simulink model "CACC_system_struct"  (Simulink 8.2)
settings: Solver=ode1  SolverMode=SingleTasking  StartTime=0.0  StopTime=inf  FixedStep=0.01  RelTol=1e-3
PreLoadFcn:
  | numd_dvsp = [0.3579 0 -0.3579];
  | dend_dvsp = [1 -1.846 0.8535];
  | simpleacc_param
PostLoadFcn:
  | , if any(exist('dsrtsu_mdlpostloadfcn', 'file') == [2, 3, 6]), try dsrtsu_mdlpostloadfcn('Execute', bdroot); catch fprintf('Error in PostLoadFcn (dsrtsu_mdlpostloadfcn) for model "%s":\n %s\n', bdroot, lasterr); end, end,
undefined symbols (not defined in the file): command_mode, max_accel_m_s2, override_enabled, speed_command_m_s, wrench_effort_command
libraries: carma_platform x3, dsrc_transmitter x2, rtitttasklib x2, lightbar x2, srx_platform x1
(part 3 of 4)

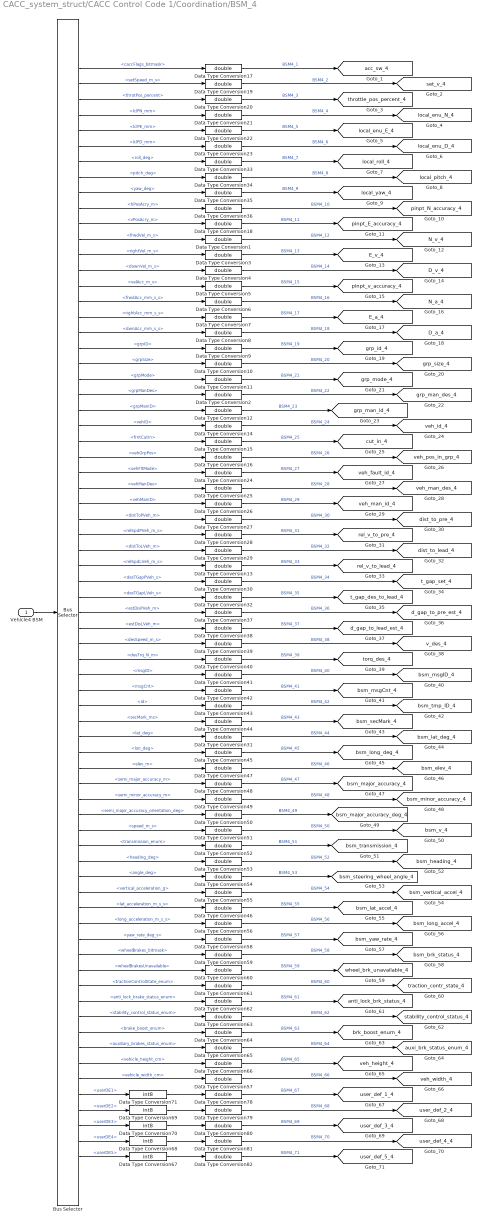
== system CACC_system_struct/CACC Control Code 1/Coordination/BSM_4 ==
  Vehicle4 BSM : Inport
  Bus Selector : BusSelector  OutputSignals=caccFlags_bitmask,setSpeed_m_s,throtPos_percent,lclPN_mm,lclPE_mm,lclPD_mm,roll_deg,pitch_deg,yaw_deg,hPosAcry_m,vPosAcry_m,frwdVel_m_s,rightVel_m_s,downVel_m_s,velAcc_m_s,frwdAcc_mm_s_s,rightAcc_mm_s_s,dwnAcc_mm_s_s,grpID,grpSize,grpMode,grpManDes,grpManID,vehID,frntCutIn,vehGrpPos,vehFltMode,vehManDes,vehManID,distToPVeh_m,relSpdPVeh_m_s,distToLVeh_m,relSpdLVeh_m_s,desTGapPVeh_s,desTGapLVeh_s,estDisPVeh_m,estDisLVeh_m,desSpeed_m_s,desTrq_N_m,msgID,msgCnt,id,secMark_ms,lat_deg,lon_deg,elev_m,semi_major_accuracy_m,semi_minor_accuracy_m,semi_major_accuracy_orientation_deg,speed_m_s,transmission_enum,heading_deg,angle_deg,vertical_acceleration_g,lat_acceleration_m_s_s,long_acceleration_m_s_s,yaw_rate_deg_s,wheelBrakes_bitmask,wheelBrakesUnavailable,tractionControlState_enum,anti_lock_brake_status_enum,stability_control_status_enum,brake_boost_enum,auxiliary_brakes_status_enum,vehicle_height_cm,vehicle_width_cm,userDE1,userDE2,userDE3,userDE4,userDE5
  Data Type Conversion{1..66,78..82} (71 alike) : DataTypeConversion  OutMin=[0]  OutMax=[5]  OutDataTypeStr=double
  Data Type Conversion{67..71} (5 alike) : DataTypeConversion  OutMin=[-128]  OutMax=[127]  OutDataTypeStr=int8  ConvertRealWorld=Stored Integer (SI)
  tag scope: D_a_4=global, D_v_4=global, E_a_4=global, E_v_4=global, N_a_4=global, N_v_4=global, acc_sw_4=global, anti_lock_brk_status_4=global, auxi_brk_status_enum_4=global, brk_boost_enum_4=global, bsm_brk_status_4=global, bsm_elev_4=global, bsm_heading_4=global, bsm_lat_accel_4=global, bsm_lat_deg_4=global, bsm_long_accel_4=global, bsm_long_deg_4=global, bsm_major_accuracy_4=global, bsm_major_accuracy_deg_4=global, bsm_minor_accuracy_4=global, bsm_msgCnt_4=global, bsm_msgID_4=global, bsm_secMark_4=global, bsm_steering_wheel_angle_4=global, bsm_tmp_ID_4=global, bsm_transmission_4=global, bsm_v_4=global, bsm_vertical_accel_4=global, bsm_yaw_rate_4=global, cut_in_4=global, d_gap_to_lead_est_4=global, d_gap_to_pre_est_4=global, dist_to_lead_4=global, dist_to_pre_4=global, grp_id_4=global, grp_man_des_4=global, grp_man_id_4=global, grp_mode_4=global, grp_size_4=global, local_enu_D_4=global, local_enu_E_4=global, local_enu_N_4=global, local_pitch_4=global, local_roll_4=global, local_yaw_4=global, pinpt_E_accuracy_4=global, pinpt_N_accuracy_4=global, pinpt_v_accuracy_4=global, rel_v_to_lead_4=global, rel_v_to_pre_4=global, set_v_4=global, stability_control_status_4=global, t_gap_des_to_lead_4=global, t_gap_set_4=global, throttle_pos_percent_4=global, torq_des_4=global, traction_contr_state_4=global, user_def_1_4=global, user_def_2_4=global, user_def_3_4=global, user_def_4_4=global, user_def_5_4=global, v_des_4=global, veh_fault_id_4=global, veh_height_4=global, veh_id_4=global, veh_man_des_4=global, veh_man_id_4=global, veh_pos_in_grp_4=global, veh_width_4=global, wheel_brk_unavailable_4=global
  wires:
  Vehicle4 BSM/1 -> Bus Selector/1
  Bus Selector/34 -> Data Type Conversion30/1  "<desTGapPVeh_s>"
  Bus Selector/33 -> Data Type Conversion13/1  "<relSpdLVeh_m_s>"
  Bus Selector/2 -> Data Type Conversion19/1  "<setSpeed_m_s>"
  Bus Selector/1 -> Data Type Conversion17/1  "<caccFlags_bitmask>"
  Bus Selector/7 -> Data Type Conversion33/1  "<roll_deg>"
  Bus Selector/3 -> Data Type Conversion20/1  "<throtPos_percent>"
  Bus Selector/9 -> Data Type Conversion35/1  "<yaw_deg>"
  Bus Selector/8 -> Data Type Conversion34/1  "<pitch_deg>"
  Bus Selector/11 -> Data Type Conversion18/1  "<vPosAcry_m>"
  Bus Selector/10 -> Data Type Conversion36/1  "<hPosAcry_m>"
  Bus Selector/13 -> Data Type Conversion3/1  "<rightVel_m_s>"
  Bus Selector/12 -> Data Type Conversion1/1  "<frwdVel_m_s>"
  Bus Selector/15 -> Data Type Conversion5/1  "<velAcc_m_s>"
  Bus Selector/14 -> Data Type Conversion4/1  "<downVel_m_s>"
  Bus Selector/17 -> Data Type Conversion7/1  "<rightAcc_mm_s_s>"
  Bus Selector/16 -> Data Type Conversion6/1  "<frwdAcc_mm_s_s>"
  Bus Selector/19 -> Data Type Conversion9/1  "<grpID>"
  Bus Selector/18 -> Data Type Conversion8/1  "<dwnAcc_mm_s_s>"
  Bus Selector/21 -> Data Type Conversion11/1  "<grpMode>"
  Bus Selector/20 -> Data Type Conversion10/1  "<grpSize>"
  Bus Selector/22 -> Data Type Conversion2/1  "<grpManDes>"
  Bus Selector/25 -> Data Type Conversion15/1  "<frntCutIn>"
  Bus Selector/24 -> Data Type Conversion14/1  "<vehID>"
  Bus Selector/27 -> Data Type Conversion24/1  "<vehFltMode>"
  Bus Selector/26 -> Data Type Conversion16/1  "<vehGrpPos>"
  Bus Selector/30 -> Data Type Conversion27/1  "<distToPVeh_m>"
  Bus Selector/29 -> Data Type Conversion26/1  "<vehManID>"
  Bus Selector/32 -> Data Type Conversion29/1  "<distToLVeh_m>"
  Bus Selector/36 -> Data Type Conversion37/1  "<estDisPVeh_m>"
  Bus Selector/35 -> Data Type Conversion32/1  "<desTGapLVeh_s>"
  Bus Selector/38 -> Data Type Conversion39/1  "<desSpeed_m_s>"
  Bus Selector/37 -> Data Type Conversion38/1  "<estDisLVeh_m>"
  Bus Selector/40 -> Data Type Conversion41/1  "<msgID>"
  Bus Selector/39 -> Data Type Conversion40/1  "<desTrq_N_m>"
  Bus Selector/42 -> Data Type Conversion43/1  "<id>"
  Bus Selector/41 -> Data Type Conversion42/1  "<msgCnt>"
  Bus Selector/44 -> Data Type Conversion31/1  "<lat_deg>"
  Bus Selector/43 -> Data Type Conversion44/1  "<secMark_ms>"
  Bus Selector/46 -> Data Type Conversion47/1  "<elev_m>"
  Bus Selector/45 -> Data Type Conversion45/1  "<lon_deg>"
  Bus Selector/48 -> Data Type Conversion49/1  "<semi_minor_accuracy_m>"
  Bus Selector/47 -> Data Type Conversion48/1  "<semi_major_accuracy_m>"
  Bus Selector/50 -> Data Type Conversion51/1  "<speed_m_s>"
  Bus Selector/49 -> Data Type Conversion50/1  "<semi_major_accuracy_orientation_deg>"
  Bus Selector/52 -> Data Type Conversion53/1  "<heading_deg>"
  Bus Selector/51 -> Data Type Conversion52/1  "<transmission_enum>"
  Bus Selector/54 -> Data Type Conversion55/1  "<vertical_acceleration_g>"
  Bus Selector/53 -> Data Type Conversion54/1  "<angle_deg>"
  Bus Selector/56 -> Data Type Conversion56/1  "<long_acceleration_m_s_s>"
  Bus Selector/55 -> Data Type Conversion46/1  "<lat_acceleration_m_s_s>"
  Bus Selector/58 -> Data Type Conversion59/1  "<wheelBrakes_bitmask>"
  Bus Selector/57 -> Data Type Conversion58/1  "<yaw_rate_deg_s>"
  Bus Selector/60 -> Data Type Conversion61/1  "<tractionControlState_enum>"
  Bus Selector/59 -> Data Type Conversion60/1  "<wheelBrakesUnavailable>"
  Bus Selector/62 -> Data Type Conversion63/1  "<stability_control_status_enum>"
  Bus Selector/61 -> Data Type Conversion62/1  "<anti_lock_brake_status_enum>"
  Bus Selector/64 -> Data Type Conversion65/1  "<auxiliary_brakes_status_enum>"
  Bus Selector/63 -> Data Type Conversion64/1  "<brake_boost_enum>"
  Bus Selector/66 -> Data Type Conversion57/1  "<vehicle_width_cm>"
  Bus Selector/65 -> Data Type Conversion66/1  "<vehicle_height_cm>"
  Bus Selector/4 -> Data Type Conversion21/1  "<lclPN_mm>"
  Bus Selector/5 -> Data Type Conversion22/1  "<lclPE_mm>"
  Bus Selector/6 -> Data Type Conversion23/1  "<lclPD_mm>"
  Bus Selector/23 -> Data Type Conversion12/1  "<grpManID>"
  Bus Selector/28 -> Data Type Conversion25/1  "<vehManDes>"
  Bus Selector/31 -> Data Type Conversion28/1  "<relSpdPVeh_m_s>"
  Bus Selector/67 -> Data Type Conversion71/1  "<userDE1>"
  Bus Selector/68 -> Data Type Conversion69/1  "<userDE2>"
  Bus Selector/69 -> Data Type Conversion70/1  "<userDE3>"
  Bus Selector/70 -> Data Type Conversion68/1  "<userDE4>"
  Bus Selector/71 -> Data Type Conversion67/1  "<userDE5>"
  Data Type Conversion66/1 -> [veh_height_4]  "BSM4_65"
  Data Type Conversion81/1 -> [user_def_4_4]  "BSM4_70"
  Data Type Conversion24/1 -> [veh_fault_id_4]  "BSM4_27"
  Data Type Conversion52/1 -> [bsm_transmission_4]  "BSM4_51"
  Data Type Conversion47/1 -> [bsm_elev_4]  "BSM4_46"
  Data Type Conversion48/1 -> [bsm_major_accuracy_4]  "BSM4_47"
  Data Type Conversion10/1 -> [grp_size_4]  "BSM4_20"
  Data Type Conversion35/1 -> [local_yaw_4]  "BSM4_9"
  Data Type Conversion59/1 -> [bsm_brk_status_4]  "BSM4_58"
  Data Type Conversion26/1 -> [veh_man_id_4]  "BSM4_29"
  Data Type Conversion42/1 -> [bsm_msgCnt_4]  "BSM4_41"
  Data Type Conversion19/1 -> [set_v_4]  "BSM4_2"
  Data Type Conversion79/1 -> [user_def_2_4]  "BSM4_68"
  Data Type Conversion27/1 -> [dist_to_pre_4]  "BSM4_30"
  Data Type Conversion2/1 -> [grp_man_des_4]  "BSM4_22"
  Data Type Conversion14/1 -> [veh_id_4]  "BSM4_24"
  Data Type Conversion9/1 -> [grp_id_4]  "BSM4_19"
  Data Type Conversion30/1 -> [t_gap_set_4]  "BSM4_34"
  Data Type Conversion32/1 -> [t_gap_des_to_lead_4]  "BSM4_35"
  Data Type Conversion31/1 -> [bsm_lat_deg_4]  "BSM4_44"
  Data Type Conversion61/1 -> [traction_contr_state_4]  "BSM4_60"
  Data Type Conversion60/1 -> [wheel_brk_unavailable_4]  "BSM4_59"
  Data Type Conversion20/1 -> [throttle_pos_percent_4]  "BSM4_3"
  Data Type Conversion36/1 -> [pinpt_N_accuracy_4]  "BSM4_10"
  Data Type Conversion78/1 -> [user_def_1_4]  "BSM4_67"
  Data Type Conversion33/1 -> [local_roll_4]  "BSM4_7"
  Data Type Conversion21/1 -> [local_enu_N_4]  "BSM4_4"
  Data Type Conversion55/1 -> [bsm_vertical_accel_4]  "BSM4_54"
  Data Type Conversion51/1 -> [bsm_v_4]  "BSM4_50"
  Data Type Conversion53/1 -> [bsm_heading_4]  "BSM4_52"
  Data Type Conversion22/1 -> [local_enu_E_4]  "BSM4_5"
  Data Type Conversion82/1 -> [user_def_5_4]  "BSM4_71"
  Data Type Conversion11/1 -> [grp_mode_4]  "BSM4_21"
  Data Type Conversion1/1 -> [N_v_4]  "BSM4_12"
  Data Type Conversion45/1 -> [bsm_long_deg_4]  "BSM4_45"
  Data Type Conversion8/1 -> [D_a_4]  "BSM4_18"
  Data Type Conversion4/1 -> [D_v_4]  "BSM4_14"
  Data Type Conversion13/1 -> [rel_v_to_lead_4]  "BSM4_33"
  Data Type Conversion62/1 -> [anti_lock_brk_status_4]  "BSM4_61"
  Data Type Conversion7/1 -> [E_a_4]  "BSM4_17"
  Data Type Conversion56/1 -> [bsm_long_accel_4]  "BSM4_56"
  Data Type Conversion80/1 -> [user_def_3_4]  "BSM4_69"
  Data Type Conversion64/1 -> [brk_boost_enum_4]  "BSM4_63"
  Data Type Conversion12/1 -> [grp_man_id_4]  "BSM4_23"
  Data Type Conversion38/1 -> [d_gap_to_lead_est_4]  "BSM4_37"
  Data Type Conversion40/1 -> [torq_des_4]  "BSM4_39"
  Data Type Conversion50/1 -> [bsm_major_accuracy_deg_4]  "BSM4_49"
  Data Type Conversion57/1 -> [veh_width_4]  "BSM4_66"
  Data Type Conversion37/1 -> [d_gap_to_pre_est_4]  "BSM4_36"
  Data Type Conversion63/1 -> [stability_control_status_4]  "BSM4_62"
  Data Type Conversion29/1 -> [dist_to_lead_4]  "BSM4_32"
  Data Type Conversion65/1 -> [auxi_brk_status_enum_4]  "BSM4_64"
  Data Type Conversion54/1 -> [bsm_steering_wheel_angle_4]  "BSM4_53"
  Data Type Conversion39/1 -> [v_des_4]  "BSM4_38"
  Data Type Conversion58/1 -> [bsm_yaw_rate_4]  "BSM4_57"
  Data Type Conversion41/1 -> [bsm_msgID_4]  "BSM4_40"
  Data Type Conversion17/1 -> [acc_sw_4]  "BSM4_1"
  Data Type Conversion28/1 -> [rel_v_to_pre_4]  "BSM4_31"
  Data Type Conversion46/1 -> [bsm_lat_accel_4]  "BSM4_55"
  Data Type Conversion5/1 -> [pinpt_v_accuracy_4]  "BSM4_15"
  Data Type Conversion15/1 -> [cut_in_4]  "BSM4_25"
  Data Type Conversion44/1 -> [bsm_secMark_4]  "BSM4_43"
  Data Type Conversion16/1 -> [veh_pos_in_grp_4]  "BSM4_26"
  Data Type Conversion34/1 -> [local_pitch_4]  "BSM4_8"
  Data Type Conversion18/1 -> [pinpt_E_accuracy_4]  "BSM4_11"
  Data Type Conversion23/1 -> [local_enu_D_4]  "BSM4_6"
  Data Type Conversion6/1 -> [N_a_4]  "BSM4_16"
  Data Type Conversion3/1 -> [E_v_4]  "BSM4_13"
  Data Type Conversion49/1 -> [bsm_minor_accuracy_4]  "BSM4_48"
  Data Type Conversion25/1 -> [veh_man_des_4]  "BSM4_28"
  Data Type Conversion43/1 -> [bsm_tmp_ID_4]  "BSM4_42"
  Data Type Conversion69/1 -> Data Type Conversion79/1
  Data Type Conversion70/1 -> Data Type Conversion80/1
  Data Type Conversion67/1 -> Data Type Conversion82/1
  Data Type Conversion71/1 -> Data Type Conversion78/1
  Data Type Conversion68/1 -> Data Type Conversion81/1

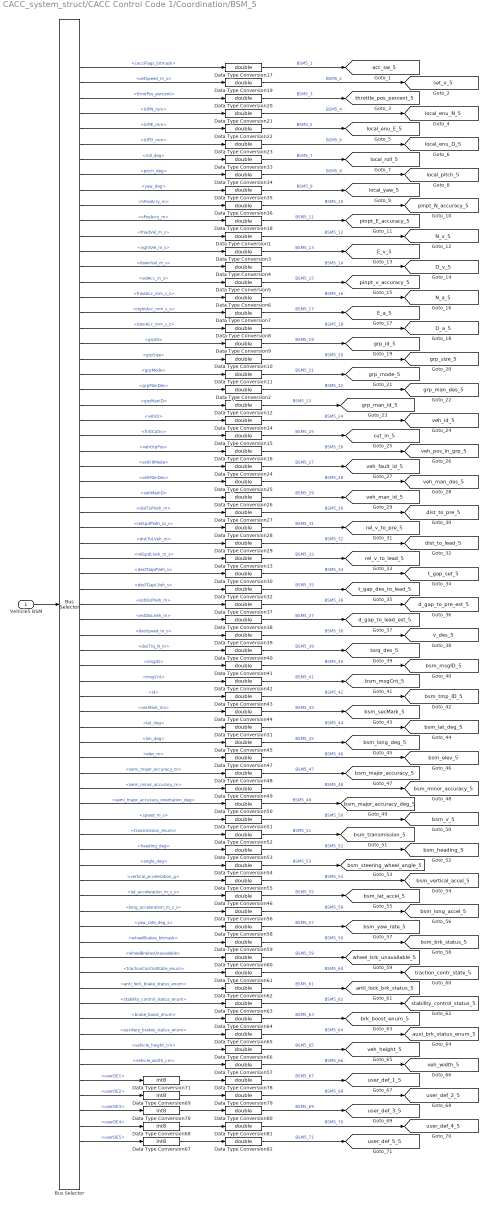
== system CACC_system_struct/CACC Control Code 1/Coordination/BSM_5 ==
  Vehicle5 BSM : Inport
  Bus Selector : BusSelector  OutputSignals=caccFlags_bitmask,setSpeed_m_s,throtPos_percent,lclPN_mm,lclPE_mm,lclPD_mm,roll_deg,pitch_deg,yaw_deg,hPosAcry_m,vPosAcry_m,frwdVel_m_s,rightVel_m_s,downVel_m_s,velAcc_m_s,frwdAcc_mm_s_s,rightAcc_mm_s_s,dwnAcc_mm_s_s,grpID,grpSize,grpMode,grpManDes,grpManID,vehID,frntCutIn,vehGrpPos,vehFltMode,vehManDes,vehManID,distToPVeh_m,relSpdPVeh_m_s,distToLVeh_m,relSpdLVeh_m_s,desTGapPVeh_s,desTGapLVeh_s,estDisPVeh_m,estDisLVeh_m,desSpeed_m_s,desTrq_N_m,msgID,msgCnt,id,secMark_ms,lat_deg,lon_deg,elev_m,semi_major_accuracy_m,semi_minor_accuracy_m,semi_major_accuracy_orientation_deg,speed_m_s,transmission_enum,heading_deg,angle_deg,vertical_acceleration_g,lat_acceleration_m_s_s,long_acceleration_m_s_s,yaw_rate_deg_s,wheelBrakes_bitmask,wheelBrakesUnavailable,tractionControlState_enum,anti_lock_brake_status_enum,stability_control_status_enum,brake_boost_enum,auxiliary_brakes_status_enum,vehicle_height_cm,vehicle_width_cm,userDE1,userDE2,userDE3,userDE4,userDE5
  Data Type Conversion{1..66,78..82} (71 alike) : DataTypeConversion  OutMin=[0]  OutMax=[5]  OutDataTypeStr=double
  Data Type Conversion{67..71} (5 alike) : DataTypeConversion  OutMin=[-128]  OutMax=[127]  OutDataTypeStr=int8  ConvertRealWorld=Stored Integer (SI)
  tag scope: D_a_5=global, D_v_5=global, E_a_5=global, E_v_5=global, N_a_5=global, N_v_5=global, acc_sw_5=global, anti_lock_brk_status_5=global, auxi_brk_status_enum_5=global, brk_boost_enum_5=global, bsm_brk_status_5=global, bsm_elev_5=global, bsm_heading_5=global, bsm_lat_accel_5=global, bsm_lat_deg_5=global, bsm_long_accel_5=global, bsm_long_deg_5=global, bsm_major_accuracy_5=global, bsm_major_accuracy_deg_5=global, bsm_minor_accuracy_5=global, bsm_msgCnt_5=global, bsm_msgID_5=global, bsm_secMark_5=global, bsm_steering_wheel_angle_5=global, bsm_tmp_ID_5=global, bsm_transmission_5=global, bsm_v_5=global, bsm_vertical_accel_5=global, bsm_yaw_rate_5=global, cut_in_5=global, d_gap_to_lead_est_5=global, d_gap_to_pre_est_5=global, dist_to_lead_5=global, dist_to_pre_5=global, grp_id_5=global, grp_man_des_5=global, grp_man_id_5=global, grp_mode_5=global, grp_size_5=global, local_enu_D_5=global, local_enu_E_5=global, local_enu_N_5=global, local_pitch_5=global, local_roll_5=global, local_yaw_5=global, pinpt_E_accuracy_5=global, pinpt_N_accuracy_5=global, pinpt_v_accuracy_5=global, rel_v_to_lead_5=global, rel_v_to_pre_5=global, set_v_5=global, stability_control_status_5=global, t_gap_des_to_lead_5=global, t_gap_set_5=global, throttle_pos_percent_5=global, torq_des_5=global, traction_contr_state_5=global, user_def_1_5=global, user_def_2_5=global, user_def_3_5=global, user_def_4_5=global, user_def_5_5=global, v_des_5=global, veh_fault_id_5=global, veh_height_5=global, veh_id_5=global, veh_man_des_5=global, veh_man_id_5=global, veh_pos_in_grp_5=global, veh_width_5=global, wheel_brk_unavailable_5=global
  wires:
  Vehicle5 BSM/1 -> Bus Selector/1
  Bus Selector/34 -> Data Type Conversion30/1  "<desTGapPVeh_s>"
  Bus Selector/33 -> Data Type Conversion13/1  "<relSpdLVeh_m_s>"
  Bus Selector/2 -> Data Type Conversion19/1  "<setSpeed_m_s>"
  Bus Selector/1 -> Data Type Conversion17/1  "<caccFlags_bitmask>"
  Bus Selector/7 -> Data Type Conversion33/1  "<roll_deg>"
  Bus Selector/3 -> Data Type Conversion20/1  "<throtPos_percent>"
  Bus Selector/9 -> Data Type Conversion35/1  "<yaw_deg>"
  Bus Selector/8 -> Data Type Conversion34/1  "<pitch_deg>"
  Bus Selector/11 -> Data Type Conversion18/1  "<vPosAcry_m>"
  Bus Selector/10 -> Data Type Conversion36/1  "<hPosAcry_m>"
  Bus Selector/13 -> Data Type Conversion3/1  "<rightVel_m_s>"
  Bus Selector/12 -> Data Type Conversion1/1  "<frwdVel_m_s>"
  Bus Selector/15 -> Data Type Conversion5/1  "<velAcc_m_s>"
  Bus Selector/14 -> Data Type Conversion4/1  "<downVel_m_s>"
  Bus Selector/17 -> Data Type Conversion7/1  "<rightAcc_mm_s_s>"
  Bus Selector/16 -> Data Type Conversion6/1  "<frwdAcc_mm_s_s>"
  Bus Selector/19 -> Data Type Conversion9/1  "<grpID>"
  Bus Selector/18 -> Data Type Conversion8/1  "<dwnAcc_mm_s_s>"
  Bus Selector/21 -> Data Type Conversion11/1  "<grpMode>"
  Bus Selector/20 -> Data Type Conversion10/1  "<grpSize>"
  Bus Selector/22 -> Data Type Conversion2/1  "<grpManDes>"
  Bus Selector/25 -> Data Type Conversion15/1  "<frntCutIn>"
  Bus Selector/24 -> Data Type Conversion14/1  "<vehID>"
  Bus Selector/27 -> Data Type Conversion24/1  "<vehFltMode>"
  Bus Selector/26 -> Data Type Conversion16/1  "<vehGrpPos>"
  Bus Selector/30 -> Data Type Conversion27/1  "<distToPVeh_m>"
  Bus Selector/29 -> Data Type Conversion26/1  "<vehManID>"
  Bus Selector/32 -> Data Type Conversion29/1  "<distToLVeh_m>"
  Bus Selector/36 -> Data Type Conversion37/1  "<estDisPVeh_m>"
  Bus Selector/35 -> Data Type Conversion32/1  "<desTGapLVeh_s>"
  Bus Selector/38 -> Data Type Conversion39/1  "<desSpeed_m_s>"
  Bus Selector/37 -> Data Type Conversion38/1  "<estDisLVeh_m>"
  Bus Selector/40 -> Data Type Conversion41/1  "<msgID>"
  Bus Selector/39 -> Data Type Conversion40/1  "<desTrq_N_m>"
  Bus Selector/42 -> Data Type Conversion43/1  "<id>"
  Bus Selector/41 -> Data Type Conversion42/1  "<msgCnt>"
  Bus Selector/44 -> Data Type Conversion31/1  "<lat_deg>"
  Bus Selector/43 -> Data Type Conversion44/1  "<secMark_ms>"
  Bus Selector/46 -> Data Type Conversion47/1  "<elev_m>"
  Bus Selector/45 -> Data Type Conversion45/1  "<lon_deg>"
  Bus Selector/48 -> Data Type Conversion49/1  "<semi_minor_accuracy_m>"
  Bus Selector/47 -> Data Type Conversion48/1  "<semi_major_accuracy_m>"
  Bus Selector/50 -> Data Type Conversion51/1  "<speed_m_s>"
  Bus Selector/49 -> Data Type Conversion50/1  "<semi_major_accuracy_orientation_deg>"
  Bus Selector/52 -> Data Type Conversion53/1  "<heading_deg>"
  Bus Selector/51 -> Data Type Conversion52/1  "<transmission_enum>"
  Bus Selector/54 -> Data Type Conversion55/1  "<vertical_acceleration_g>"
  Bus Selector/53 -> Data Type Conversion54/1  "<angle_deg>"
  Bus Selector/56 -> Data Type Conversion56/1  "<long_acceleration_m_s_s>"
  Bus Selector/55 -> Data Type Conversion46/1  "<lat_acceleration_m_s_s>"
  Bus Selector/58 -> Data Type Conversion59/1  "<wheelBrakes_bitmask>"
  Bus Selector/57 -> Data Type Conversion58/1  "<yaw_rate_deg_s>"
  Bus Selector/60 -> Data Type Conversion61/1  "<tractionControlState_enum>"
  Bus Selector/59 -> Data Type Conversion60/1  "<wheelBrakesUnavailable>"
  Bus Selector/62 -> Data Type Conversion63/1  "<stability_control_status_enum>"
  Bus Selector/61 -> Data Type Conversion62/1  "<anti_lock_brake_status_enum>"
  Bus Selector/64 -> Data Type Conversion65/1  "<auxiliary_brakes_status_enum>"
  Bus Selector/63 -> Data Type Conversion64/1  "<brake_boost_enum>"
  Bus Selector/66 -> Data Type Conversion57/1  "<vehicle_width_cm>"
  Bus Selector/65 -> Data Type Conversion66/1  "<vehicle_height_cm>"
  Bus Selector/4 -> Data Type Conversion21/1  "<lclPN_mm>"
  Bus Selector/5 -> Data Type Conversion22/1  "<lclPE_mm>"
  Bus Selector/6 -> Data Type Conversion23/1  "<lclPD_mm>"
  Bus Selector/23 -> Data Type Conversion12/1  "<grpManID>"
  Bus Selector/28 -> Data Type Conversion25/1  "<vehManDes>"
  Bus Selector/31 -> Data Type Conversion28/1  "<relSpdPVeh_m_s>"
  Bus Selector/67 -> Data Type Conversion71/1  "<userDE1>"
  Bus Selector/68 -> Data Type Conversion69/1  "<userDE2>"
  Bus Selector/69 -> Data Type Conversion70/1  "<userDE3>"
  Bus Selector/70 -> Data Type Conversion68/1  "<userDE4>"
  Bus Selector/71 -> Data Type Conversion67/1  "<userDE5>"
  Data Type Conversion63/1 -> [stability_control_status_5]  "BSM5_62"
  Data Type Conversion78/1 -> [user_def_1_5]  "BSM5_67"
  Data Type Conversion5/1 -> [pinpt_v_accuracy_5]  "BSM5_15"
  Data Type Conversion64/1 -> [brk_boost_enum_5]  "BSM5_63"
  Data Type Conversion26/1 -> [veh_man_id_5]  "BSM5_29"
  Data Type Conversion56/1 -> [bsm_long_accel_5]  "BSM5_56"
  Data Type Conversion62/1 -> [anti_lock_brk_status_5]  "BSM5_61"
  Data Type Conversion53/1 -> [bsm_heading_5]  "BSM5_52"
  Data Type Conversion33/1 -> [local_roll_5]  "BSM5_7"
  Data Type Conversion79/1 -> [user_def_2_5]  "BSM5_68"
  Data Type Conversion42/1 -> [bsm_msgCnt_5]  "BSM5_41"
  Data Type Conversion24/1 -> [veh_fault_id_5]  "BSM5_27"
  Data Type Conversion14/1 -> [veh_id_5]  "BSM5_24"
  Data Type Conversion61/1 -> [traction_contr_state_5]  "BSM5_60"
  Data Type Conversion9/1 -> [grp_id_5]  "BSM5_19"
  Data Type Conversion66/1 -> [veh_height_5]  "BSM5_65"
  Data Type Conversion80/1 -> [user_def_3_5]  "BSM5_69"
  Data Type Conversion65/1 -> [auxi_brk_status_enum_5]  "BSM5_64"
  Data Type Conversion4/1 -> [D_v_5]  "BSM5_14"
  Data Type Conversion82/1 -> [user_def_5_5]  "BSM5_71"
  Data Type Conversion1/1 -> [N_v_5]  "BSM5_12"
  Data Type Conversion38/1 -> [d_gap_to_lead_est_5]  "BSM5_37"
  Data Type Conversion54/1 -> [bsm_steering_wheel_angle_5]  "BSM5_53"
  Data Type Conversion55/1 -> [bsm_vertical_accel_5]  "BSM5_54"
  Data Type Conversion44/1 -> [bsm_secMark_5]  "BSM5_43"
  Data Type Conversion6/1 -> [N_a_5]  "BSM5_16"
  Data Type Conversion7/1 -> [E_a_5]  "BSM5_17"
  Data Type Conversion60/1 -> [wheel_brk_unavailable_5]  "BSM5_59"
  Data Type Conversion3/1 -> [E_v_5]  "BSM5_13"
  Data Type Conversion50/1 -> [bsm_major_accuracy_deg_5]  "BSM5_49"
  Data Type Conversion52/1 -> [bsm_transmission_5]  "BSM5_51"
  Data Type Conversion8/1 -> [D_a_5]  "BSM5_18"
  Data Type Conversion32/1 -> [t_gap_des_to_lead_5]  "BSM5_35"
  Data Type Conversion49/1 -> [bsm_minor_accuracy_5]  "BSM5_48"
  Data Type Conversion21/1 -> [local_enu_N_5]  "BSM5_4"
  Data Type Conversion17/1 -> [acc_sw_5]  "BSM5_1"
  Data Type Conversion81/1 -> [user_def_4_5]  "BSM5_70"
  Data Type Conversion51/1 -> [bsm_v_5]  "BSM5_50"
  Data Type Conversion46/1 -> [bsm_lat_accel_5]  "BSM5_55"
  Data Type Conversion59/1 -> [bsm_brk_status_5]  "BSM5_58"
  Data Type Conversion11/1 -> [grp_mode_5]  "BSM5_21"
  Data Type Conversion47/1 -> [bsm_elev_5]  "BSM5_46"
  Data Type Conversion18/1 -> [pinpt_E_accuracy_5]  "BSM5_11"
  Data Type Conversion16/1 -> [veh_pos_in_grp_5]  "BSM5_26"
  Data Type Conversion2/1 -> [grp_man_des_5]  "BSM5_22"
  Data Type Conversion57/1 -> [veh_width_5]  "BSM5_66"
  Data Type Conversion45/1 -> [bsm_long_deg_5]  "BSM5_45"
  Data Type Conversion40/1 -> [torq_des_5]  "BSM5_39"
  Data Type Conversion43/1 -> [bsm_tmp_ID_5]  "BSM5_42"
  Data Type Conversion48/1 -> [bsm_major_accuracy_5]  "BSM5_47"
  Data Type Conversion41/1 -> [bsm_msgID_5]  "BSM5_40"
  Data Type Conversion58/1 -> [bsm_yaw_rate_5]  "BSM5_57"
  Data Type Conversion10/1 -> [grp_size_5]  "BSM5_20"
  Data Type Conversion15/1 -> [cut_in_5]  "BSM5_25"
  Data Type Conversion27/1 -> [dist_to_pre_5]  "BSM5_30"
  Data Type Conversion12/1 -> [grp_man_id_5]  "BSM5_23"
  Data Type Conversion37/1 -> [d_gap_to_pre_est_5]  "BSM5_36"
  Data Type Conversion31/1 -> [bsm_lat_deg_5]  "BSM5_44"
  Data Type Conversion19/1 -> [set_v_5]  "BSM5_2"
  Data Type Conversion20/1 -> [throttle_pos_percent_5]  "BSM5_3"
  Data Type Conversion13/1 -> [rel_v_to_lead_5]  "BSM5_33"
  Data Type Conversion39/1 -> [v_des_5]  "BSM5_38"
  Data Type Conversion35/1 -> [local_yaw_5]  "BSM5_9"
  Data Type Conversion30/1 -> [t_gap_set_5]  "BSM5_34"
  Data Type Conversion36/1 -> [pinpt_N_accuracy_5]  "BSM5_10"
  Data Type Conversion22/1 -> [local_enu_E_5]  "BSM5_5"
  Data Type Conversion25/1 -> [veh_man_des_5]  "BSM5_28"
  Data Type Conversion23/1 -> [local_enu_D_5]  "BSM5_6"
  Data Type Conversion28/1 -> [rel_v_to_pre_5]  "BSM5_31"
  Data Type Conversion29/1 -> [dist_to_lead_5]  "BSM5_32"
  Data Type Conversion34/1 -> [local_pitch_5]  "BSM5_8"
  Data Type Conversion71/1 -> Data Type Conversion78/1
  Data Type Conversion69/1 -> Data Type Conversion79/1
  Data Type Conversion68/1 -> Data Type Conversion81/1
  Data Type Conversion70/1 -> Data Type Conversion80/1
  Data Type Conversion67/1 -> Data Type Conversion82/1

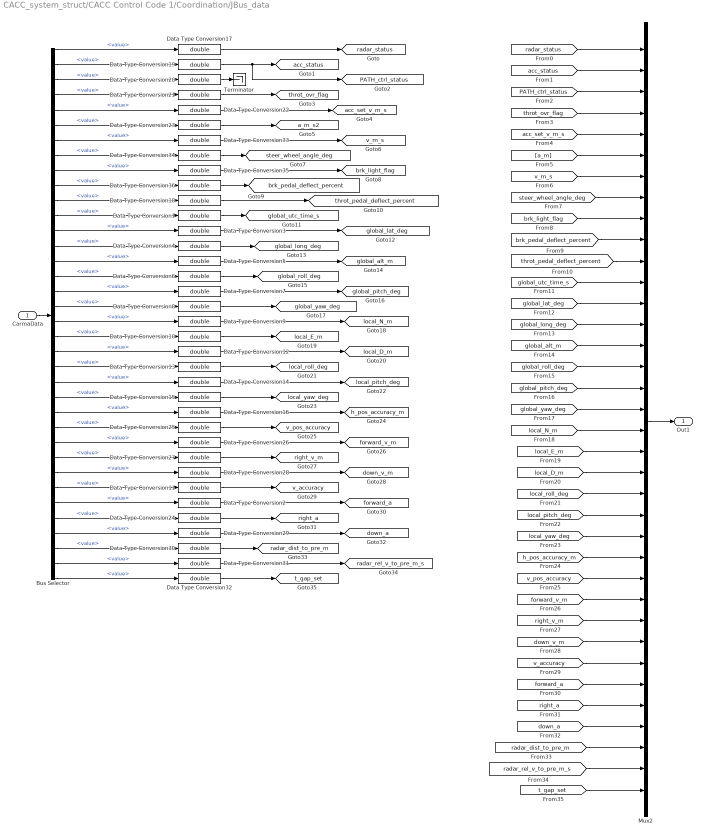
== system CACC_system_struct/CACC Control Code 1/Coordination/JBus_data ==
  CarmaData : Inport
  Bus Selector : BusSelector  OutputSignals=radar_status.value,acc_status.value,path_ctrl_status.value,throttle_ovr_flag.value,acc_set_speed_m_s.value,accel_m_s2.value,speed_m_s.value,steering_wheel_angle_deg.value,brk_light_flag.value,brk_pedal_deflect_percent.value,throttle_pedal_deflect_percent.value,global_utc_time_s.value,global_lat_deg.value,global_long_deg.value,global_alt_m.value,global_roll_deg.value,global_pitch_deg.value,global_yaw_deg.value,local_north_m.value,local_east_m.value,local_down_m.value,local_roll_deg.value,local_pitch_deg.value,local_yaw_deg.value,horizontal_pos_accuracy_m.value,vertical_pos_accuracy_m.value,velocity_fwd_m_s.value,velocity_right_m_s.value,velocity_down_m_s.value,velocity_accuracy_m_s.value,accel_fwd_m_s2.value,accel_right_m_s2.value,accel_down_m_s2.value,dist_to_preceding_veh_m.value,rel_speed_to_preceding_veh_m_s.value,desired_headway.value
  Data Type Conversion{1..36} (36 alike) : DataTypeConversion  OutMin=[0]  OutMax=[5]  OutDataTypeStr=double
  Mux2 : Mux  Inputs=36
  Terminator : Terminator
  Out1 : Outport
  tag scope: PATH_ctrl_status=global, a_m_s2=global, acc_set_v_m_s=global, acc_status=global, brk_light_flag=global, brk_pedal_deflect_percent=global, down_a=global, down_v_m=global, forward_a=global, forward_v_m=global, global_alt_m=global, global_lat_deg=global, global_long_deg=global, global_pitch_deg=global, global_roll_deg=global, global_utc_time_s=global, global_yaw_deg=global, h_pos_accuracy_m=global, local_D_m=global, local_E_m=global, local_N_m=global, local_pitch_deg=global, local_roll_deg=global, local_yaw_deg=global, radar_dist_to_pre_m=global, radar_rel_v_to_pre_m_s=global, radar_status=global, right_a=global, right_v_m=global, steer_wheel_angle_deg=global, t_gap_set=global, throt_ovr_flag=global, throt_pedal_deflect_percent=global, v_accuracy=global, v_m_s=global, v_pos_accuracy=global
  wires:
  Mux2/1 -> Out1/1
  [acc_status] -> Mux2/2
  [throt_ovr_flag] -> Mux2/4
  [a_m] -> Mux2/6
  [steer_wheel_angle_deg] -> Mux2/8
  [brk_pedal_deflect_percent] -> Mux2/10
  [global_utc_time_s] -> Mux2/12
  [global_long_deg] -> Mux2/14
  [radar_status] -> Mux2/1
  [PATH_ctrl_status] -> Mux2/3
  [acc_set_v_m_s] -> Mux2/5
  [v_m_s] -> Mux2/7
  [brk_light_flag] -> Mux2/9
  [throt_pedal_deflect_percent] -> Mux2/11
  [global_lat_deg] -> Mux2/13
  [global_alt_m] -> Mux2/15
  [global_roll_deg] -> Mux2/16
  [global_yaw_deg] -> Mux2/18
  [global_pitch_deg] -> Mux2/17
  [local_N_m] -> Mux2/19
  [local_D_m] -> Mux2/21
  [local_E_m] -> Mux2/20
  [local_roll_deg] -> Mux2/22
  [local_pitch_deg] -> Mux2/23
  [h_pos_accuracy_m] -> Mux2/25
  [local_yaw_deg] -> Mux2/24
  [v_pos_accuracy] -> Mux2/26
  [right_v_m] -> Mux2/28
  [forward_v_m] -> Mux2/27
  [down_v_m] -> Mux2/29
  [v_accuracy] -> Mux2/30
  [right_a] -> Mux2/32
  [forward_a] -> Mux2/31
  [down_a] -> Mux2/33
  [radar_dist_to_pre_m] -> Mux2/34
  [radar_rel_v_to_pre_m_s] -> Mux2/35
  [t_gap_set] -> Mux2/36
  Bus Selector/1 -> Data Type Conversion17/1  "<value>"
  Bus Selector/2 -> Data Type Conversion19/1  "<value>"
  Bus Selector/3 -> Data Type Conversion20/1  "<value>"
  Bus Selector/4 -> Data Type Conversion21/1  "<value>"
  Bus Selector/5 -> Data Type Conversion22/1  "<value>"
  Bus Selector/6 -> Data Type Conversion23/1  "<value>"
  Bus Selector/7 -> Data Type Conversion33/1  "<value>"
  Bus Selector/8 -> Data Type Conversion34/1  "<value>"
  Bus Selector/9 -> Data Type Conversion35/1  "<value>"
  Bus Selector/10 -> Data Type Conversion36/1  "<value>"
  Bus Selector/11 -> Data Type Conversion18/1  "<value>"
  Bus Selector/12 -> Data Type Conversion1/1  "<value>"
  Bus Selector/13 -> Data Type Conversion3/1  "<value>"
  Bus Selector/14 -> Data Type Conversion4/1  "<value>"
  Bus Selector/15 -> Data Type Conversion5/1  "<value>"
  Bus Selector/16 -> Data Type Conversion6/1  "<value>"
  Bus Selector/17 -> Data Type Conversion7/1  "<value>"
  Bus Selector/18 -> Data Type Conversion8/1  "<value>"
  Bus Selector/19 -> Data Type Conversion9/1  "<value>"
  Bus Selector/20 -> Data Type Conversion10/1  "<value>"
  Bus Selector/21 -> Data Type Conversion12/1  "<value>"
  Bus Selector/22 -> Data Type Conversion13/1  "<value>"
  Bus Selector/23 -> Data Type Conversion14/1  "<value>"
  Bus Selector/24 -> Data Type Conversion15/1  "<value>"
  Bus Selector/25 -> Data Type Conversion16/1  "<value>"
  Bus Selector/26 -> Data Type Conversion25/1  "<value>"
  Bus Selector/27 -> Data Type Conversion26/1  "<value>"
  Bus Selector/28 -> Data Type Conversion27/1  "<value>"
  Bus Selector/29 -> Data Type Conversion28/1  "<value>"
  Bus Selector/30 -> Data Type Conversion11/1  "<value>"
  Bus Selector/31 -> Data Type Conversion2/1  "<value>"
  Bus Selector/32 -> Data Type Conversion24/1  "<value>"
  Bus Selector/33 -> Data Type Conversion29/1  "<value>"
  Bus Selector/34 -> Data Type Conversion30/1  "<value>"
  Bus Selector/35 -> Data Type Conversion31/1  "<value>"
  Bus Selector/36 -> Data Type Conversion32/1  "<value>"
  Data Type Conversion17/1 -> [radar_status]
  Data Type Conversion19/1 -> [PATH_ctrl_status], [acc_status]
  Data Type Conversion21/1 -> [throt_ovr_flag]
  Data Type Conversion22/1 -> [acc_set_v_m_s]
  Data Type Conversion23/1 -> [a_m_s2]
  Data Type Conversion33/1 -> [v_m_s]
  Data Type Conversion34/1 -> [steer_wheel_angle_deg]
  Data Type Conversion35/1 -> [brk_light_flag]
  Data Type Conversion36/1 -> [brk_pedal_deflect_percent]
  Data Type Conversion18/1 -> [throt_pedal_deflect_percent]
  Data Type Conversion1/1 -> [global_utc_time_s]
  Data Type Conversion3/1 -> [global_lat_deg]
  Data Type Conversion4/1 -> [global_long_deg]
  Data Type Conversion5/1 -> [global_alt_m]
  Data Type Conversion6/1 -> [global_roll_deg]
  Data Type Conversion7/1 -> [global_pitch_deg]
  Data Type Conversion8/1 -> [global_yaw_deg]
  Data Type Conversion9/1 -> [local_N_m]
  Data Type Conversion13/1 -> [local_roll_deg]
  Data Type Conversion15/1 -> [local_yaw_deg]
  Data Type Conversion16/1 -> [h_pos_accuracy_m]
  Data Type Conversion25/1 -> [v_pos_accuracy]
  Data Type Conversion26/1 -> [forward_v_m]
  Data Type Conversion24/1 -> [right_a]
  Data Type Conversion2/1 -> [forward_a]
  Data Type Conversion27/1 -> [right_v_m]
  Data Type Conversion10/1 -> [local_E_m]
  Data Type Conversion11/1 -> [v_accuracy]
  Data Type Conversion30/1 -> [radar_dist_to_pre_m]
  Data Type Conversion28/1 -> [down_v_m]
  Data Type Conversion31/1 -> [radar_rel_v_to_pre_m_s]
  Data Type Conversion14/1 -> [local_pitch_deg]
  Data Type Conversion12/1 -> [local_D_m]
  Data Type Conversion32/1 -> [t_gap_set]
  Data Type Conversion29/1 -> [down_a]
  Data Type Conversion20/1 -> Terminator/1
  CarmaData/1 -> Bus Selector/1

== system CACC_system_struct/CACC Control Code 1/Coordination/Subj_veh_info ==
  Out1 : Outport
  wires:
  [subj_veh_id] -> Out1/1

== system CACC_system_struct/CACC Control Code 1/Coordination/Veh Pos Input ==
  Mux2 : Mux  Inputs=15
  Out1 : Outport
  wires:
  Mux2/1 -> Out1/1
  [BSM1_id] -> Mux2/1
  [BSM1_control_pos] -> Mux2/2
  [BSM1_lane_id] -> Mux2/3
  [BSM2_id] -> Mux2/4
  [BSM2_control_pos] -> Mux2/5
  [BSM2_lane_id] -> Mux2/6
  [BSM3_id] -> Mux2/7
  [BSM3_control_pos] -> Mux2/8
  [BSM3_lane_id] -> Mux2/9
  [BSM4_id] -> Mux2/10
  [BSM4_control_pos] -> Mux2/11
  [BSM4_lane_id] -> Mux2/12
  [BSM5_id] -> Mux2/13
  [BSM5_control_pos] -> Mux2/14
  [BSM5_lane_id] -> Mux2/15

== system CACC_system_struct/CACC Control Code 1/Coordination/Veh Pos Output ==
  In1 : Inport
  Demux : Demux  Outputs=15
  tag scope: BSM1_control_pos=global, BSM1_id=global, BSM1_lane_id=global, BSM2_control_pos=global, BSM2_id=global, BSM2_lane_id=global, BSM3_control_pos=global, BSM3_id=global, BSM3_lane_id=global, BSM4_control_pos=global, BSM4_id=global, BSM4_lane_id=global, BSM5_control_pos=global, BSM5_id=global, BSM5_lane_id=global
  wires:
  In1/1 -> Demux/1
  Demux/1 -> [BSM1_id]  "BMS1_id"
  Demux/2 -> [BSM1_control_pos]  "BSM1_control_pos"
  Demux/3 -> [BSM1_lane_id]  "BMS1_lane_id"
  Demux/4 -> [BSM2_id]  "BMS2_id"
  Demux/5 -> [BSM2_control_pos]  "BSM2_control_pos"
  Demux/6 -> [BSM2_lane_id]  "BMS2_lane_id"
  Demux/7 -> [BSM3_id]  "BSM3_id"
  Demux/8 -> [BSM3_control_pos]  "BSM3_control_pos"
  Demux/9 -> [BSM3_lane_id]  "BSM3_lane_id"
  Demux/10 -> [BSM4_id]  "BSM4_id"
  Demux/11 -> [BSM4_control_pos]  "BSM4_control_pos"
  Demux/12 -> [BSM4_lane_id]  "BSM4_lane_id"
  Demux/13 -> [BSM5_id]  "BSM5_id"
  Demux/14 -> [BSM5_control_pos]  "BSM5_control_pos"
  Demux/15 -> [BSM5_lane_id]  "BSM5_lane_id"

== system CACC_system_struct/CACC Control Code 1/Coordination/lead_veh ==
  In1 : Inport
  Demux : Demux  Outputs=17
  tag scope: lead_a=global, lead_a_des=global, lead_acc_sw=global, lead_brk_pedal_deflect=global, lead_cacc_sw=global, lead_control_pos=global, lead_d=global, lead_d_ref=global, lead_drive_mode=global, lead_fault_mode=global, lead_man_des=global, lead_radar_range=global, lead_radar_rate=global, lead_run_flag=global, lead_v=global, lead_v_des=global, lead_v_ref=global
  wires:
  In1/1 -> Demux/1
  Demux/1 -> [lead_acc_sw]
  Demux/2 -> [lead_cacc_sw]
  Demux/3 -> [lead_fault_mode]
  Demux/4 -> [lead_control_pos]
  Demux/5 -> [lead_drive_mode]
  Demux/6 -> [lead_man_des]
  Demux/7 -> [lead_a]
  Demux/8 -> [lead_v]
  Demux/9 -> [lead_d]
  Demux/10 -> [lead_v_ref]
  Demux/11 -> [lead_d_ref]
  Demux/12 -> [lead_radar_range]
  Demux/13 -> [lead_radar_rate]
  Demux/14 -> [lead_brk_pedal_deflect]
  Demux/15 -> [lead_v_des]
  Demux/16 -> [lead_a_des]
  Demux/17 -> [lead_run_flag]

== system CACC_system_struct/CACC Control Code 1/Coordination/pre_veh ==
  In1 : Inport
  Demux : Demux  Outputs=17
  tag scope: pre_a=global, pre_a_des=global, pre_acc_sw=global, pre_brk_pedal_deflect=global, pre_cacc_sw=global, pre_control_pos=global, pre_d=global, pre_d_ref=global, pre_drive_mode=global, pre_fault_mode=global, pre_man_des=global, pre_radar_range=global, pre_radar_rate=global, pre_run_flag=global, pre_v=global, pre_v_des=global, pre_v_ref=global
  wires:
  In1/1 -> Demux/1
  Demux/1 -> [pre_acc_sw]
  Demux/2 -> [pre_cacc_sw]
  Demux/3 -> [pre_fault_mode]
  Demux/4 -> [pre_control_pos]
  Demux/5 -> [pre_drive_mode]
  Demux/6 -> [pre_man_des]
  Demux/7 -> [pre_a]
  Demux/8 -> [pre_v]
  Demux/9 -> [pre_d]
  Demux/10 -> [pre_v_ref]
  Demux/11 -> [pre_d_ref]
  Demux/12 -> [pre_radar_range]
  Demux/13 -> [pre_radar_rate]
  Demux/14 -> [pre_brk_pedal_deflect]
  Demux/15 -> [pre_v_des]
  Demux/16 -> [pre_a_des]
  Demux/17 -> [pre_run_flag]

== system CACC_system_struct/CACC Control Code 1/Coordination/subj_veh ==
  In1 : Inport
  Demux : Demux  Outputs=26
  Terminator : Terminator
  Terminator1 : Terminator
  tag scope: Emergent_brk_flag=global, control_pos=global, cut_in_flag=global, des_d_gap_to_lead=global, des_d_gap_to_pre=global, drive_mode=global, dsrc_status=global, global_synch_t=global, grp_id=global, grp_man_des=global, grp_man_id=global, grp_mode=global, grp_size=global, man_des=global, man_id=global, rel_d_to_lead_est=global, rel_d_to_pre=global, rel_v_to_lead_est=global, rel_v_to_pre=global, user_def_1=global, user_def_2=global, user_def_3=global, user_def_4=global, user_def_5=global, veh_fault_id=global, veh_id=global
  wires:
  In1/1 -> Demux/1
  Demux/1 -> [global_synch_t]
  Demux/2 -> [grp_id]
  Demux/3 -> [grp_size]
  Demux/4 -> [grp_mode]
  Demux/5 -> [grp_man_des]
  Demux/6 -> [grp_man_id]
  Demux/7 -> [veh_id]
  Demux/8 -> [dsrc_status]
  Demux/9 -> [veh_fault_id]
  Demux/10 -> [cut_in_flag]
  Demux/11 -> [control_pos]
  Demux/12 -> [man_des]
  Demux/13 -> [man_id]
  Demux/14 -> [drive_mode]
  Demux/15 -> Terminator1/1
  Demux/16 -> Terminator/1
  Demux/17 -> [rel_v_to_lead_est]
  Demux/18 -> [rel_d_to_lead_est]
  Demux/19 -> [des_d_gap_to_pre]
  Demux/20 -> [des_d_gap_to_lead]
  Demux/21 -> [Emergent_brk_flag]
  Demux/22 -> [user_def_1]
  Demux/23 -> [user_def_2]
  Demux/24 -> [user_def_3]
  Demux/25 -> [user_def_4]
  Demux/26 -> [user_def_5]
  [radar_rel_v_to_pre_m_s] -> [rel_v_to_pre]
  [radar_dist_to_pre_m] -> [rel_d_to_pre]

== system CACC_system_struct/CACC Control Code 1/Ethernet TX - to DSRC/Subj_Veh_Msg_to_Memory_Store ==
  Constant : Constant
  Constant1 : Constant  Value=100
  Data Type Conversion{10..16,18..22,24,27,29,31..36} (21 alike) : DataTypeConversion  OutMin=[0]  OutMax=[5]  OutDataTypeStr=uint8
  Data Type Conversion{23,25..26,28} (4 alike) : DataTypeConversion  OutMin=[0]  OutMax=[5]  OutDataTypeStr=single
  Data Type Conversion30 : DataTypeConversion  OutMin=[0]  OutMax=[5]  OutDataTypeStr=uint16
  Demux : Demux  Outputs=26
  Divide : Product  Inputs=*/
  MinMax : MinMax  Function=max  Inputs=2
  Mux2 : Mux  Inputs=26
  Product13 : Product
  Terminator : Terminator
  Terminator1 : Terminator
  Terminator2 : Terminator
  Update Current BSM Data : Subsystem
  CACC Data : Outport
  wires:
  Mux2/1 -> [BSM_Memory_Store]
  [v_des] -> Mux2/20
  [des_d_gap_to_lead] -> Mux2/19
  [des_d_gap_to_pre] -> Mux2/18
  [des_t_gap_to_lead] -> Mux2/17
  [rel_v_to_lead_est] -> Mux2/15
  [rel_v_to_pre] -> Mux2/13
  [rel_d_to_pre] -> Mux2/12
  [man_id] -> Mux2/11
  [man_des] -> Mux2/10
  [veh_fault_id] -> Mux2/9
  [control_pos] -> Mux2/8
  [grp_id] -> Mux2/1
  [grp_size] -> Mux2/2
  [grp_mode] -> Mux2/3
  [grp_man_des] -> Mux2/4
  [grp_man_id] -> Mux2/5
  [veh_id] -> Mux2/6
  [cut_in_flag] -> Mux2/7
  [rel_d_to_lead_est] -> Mux2/14
  [t_gap_set] -> Mux2/16
  [user_def_5] -> Mux2/26
  [user_def_4] -> Mux2/25
  [usyn] -> Mux2/24
  [drive_mode] -> Mux2/23
  [run_flag] -> Mux2/22
  [BSM_Memory_Store] -> Demux/1
  Demux/1 -> Data Type Conversion24/1
  Demux/2 -> Data Type Conversion10/1
  Demux/3 -> Data Type Conversion11/1
  Demux/4 -> Data Type Conversion14/1
  Demux/5 -> Data Type Conversion12/1
  Demux/6 -> Data Type Conversion13/1
  Demux/7 -> Data Type Conversion18/1
  Demux/8 -> Data Type Conversion15/1
  Demux/9 -> Data Type Conversion16/1
  Demux/10 -> Data Type Conversion21/1
  Demux/11 -> Data Type Conversion19/1
  Demux/12 -> Data Type Conversion20/1
  Demux/13 -> Data Type Conversion25/1
  Demux/14 -> Data Type Conversion22/1
  Demux/15 -> Data Type Conversion23/1
  Demux/16 -> Data Type Conversion28/1
  Demux/17 -> Data Type Conversion26/1
  Demux/18 -> Data Type Conversion27/1
  Demux/19 -> Data Type Conversion31/1
  Demux/20 -> Data Type Conversion29/1
  Demux/21 -> Data Type Conversion30/1
  Demux/22 -> Data Type Conversion34/1
  Demux/23 -> Data Type Conversion32/1
  Demux/24 -> Data Type Conversion33/1
  Demux/25 -> Data Type Conversion35/1
  Demux/26 -> Data Type Conversion36/1
  Data Type Conversion24/1 -> Update Current BSM Data/1(grpID)
  Data Type Conversion10/1 -> Update Current BSM Data/2(grpSize)
  Data Type Conversion11/1 -> Update Current BSM Data/3(grpMode)
  Data Type Conversion13/1 -> Update Current BSM Data/6(vehID)
  Data Type Conversion12/1 -> Update Current BSM Data/5(grpManID)
  Data Type Conversion14/1 -> Update Current BSM Data/4(grpManDes)
  Data Type Conversion18/1 -> Update Current BSM Data/7(frntCutIn)
  Data Type Conversion16/1 -> Update Current BSM Data/9(vehFltMode)
  Data Type Conversion15/1 -> Update Current BSM Data/8(vehGrpPos)
  Data Type Conversion21/1 -> Update Current BSM Data/10(vehManDes)
  Data Type Conversion19/1 -> Update Current BSM Data/11(vehManID)
  Data Type Conversion20/1 -> Update Current BSM Data/12(distToPVeh_m)
  Data Type Conversion25/1 -> Update Current BSM Data/13(relSpdPVeh_m_s)
  Data Type Conversion23/1 -> Update Current BSM Data/15(relSpdLVeh_m_s)
  Data Type Conversion26/1 -> Update Current BSM Data/17(desTGapLVeh_s)
  Data Type Conversion27/1 -> Update Current BSM Data/18(estDisPVeh_m)
  Data Type Conversion28/1 -> Update Current BSM Data/16(desTGapPVeh_s)
  Data Type Conversion29/1 -> Update Current BSM Data/20(desSpeed_m_s)
  Data Type Conversion30/1 -> Update Current BSM Data/21(desTrq_N_m)
  Data Type Conversion31/1 -> Update Current BSM Data/19(estDisLVeh_m)
  Data Type Conversion32/1 -> Update Current BSM Data/23(userDE2)
  Data Type Conversion34/1 -> Update Current BSM Data/22(userDE1)
  Data Type Conversion33/1 -> Update Current BSM Data/24(userDE3)
  Data Type Conversion35/1 -> Update Current BSM Data/25(userDE4)
  Data Type Conversion36/1 -> Update Current BSM Data/26(userDE5)
  Data Type Conversion22/1 -> Update Current BSM Data/14(distToLVeh_m_s)
  Update Current BSM Data/1(CACC Data) -> CACC Data/1
  [des_d_gap_to_lead] -> Divide/1
  [v_des] -> MinMax/1
  Constant/1 -> MinMax/2
  Divide/1 -> [des_t_gap_to_lead]
  MinMax/1 -> Divide/2
  [user_def_1] -> Terminator/1
  [user_def_3] -> Terminator2/1
  [user_def_2] -> Terminator1/1
  [usyn] -> Product13/1
  Constant1/1 -> Product13/2
  Product13/1 -> Mux2/21

== system CACC_system_struct/RTI Data/RTI Data Store/RTI Data Store ==
  RTI Data Store : Subsystem  mask(RTI_DATA_STORE){}
      mask help:
      | RTI Data Store Block. This block is used by RTI to store internal model dependent data. Deleting this block will result in data loss.
      |
      | NEVER DELETE, COPY, OR MODIFY THIS BLOCK!
      mask Help:
      | RTI Data Store Block. This block is used by RTI to store internal model dependent data. Deleting this block will result in data loss.
      | 
      | NEVER DELETE, COPY, OR MODIFY THIS BLOCK!
      mask Display: text(0.5, 0.5, ' ', 'HorizontalAlignment', 'center');

== system CACC_system_struct/CACC Control Code 1/Ethernet TX - to DSRC/Subj_Veh_Msg_to_Memory_Store/Update Current BSM Data ==
  grpID : Inport
  grpSize : Inport  Port=2
  grpMode : Inport  Port=3
  grpManDes : Inport  Port=4
  grpManID : Inport  Port=5
  vehID : Inport  Port=6
  frntCutIn : Inport  Port=7
  vehGrpPos : Inport  Port=8
  vehFltMode : Inport  Port=9
  vehManDes : Inport  Port=10
  vehManID : Inport  Port=11
  distToPVeh_m : Inport  Port=12
  relSpdPVeh_m_s : Inport  Port=13
  distToLVeh_m_s : Inport  Port=14
  relSpdLVeh_m_s : Inport  Port=15
  desTGapPVeh_s : Inport  Port=16
  desTGapLVeh_s : Inport  Port=17
  estDisPVeh_m : Inport  Port=18
  estDisLVeh_m : Inport  Port=19
  desSpeed_m_s : Inport  Port=20
  desTrq_N_m : Inport  Port=21
  userDE1 : Inport  Port=22
  userDE2 : Inport  Port=23
  userDE3 : Inport  Port=24
  userDE4 : Inport  Port=25
  userDE5 : Inport  Port=26
  Bus Creator : BusCreator  Inputs=26
  CACC Data : Outport
  wires:
  Bus Creator/1 -> CACC Data/1
  userDE5/1 -> Bus Creator/26
  userDE4/1 -> Bus Creator/25
  userDE3/1 -> Bus Creator/24
  userDE2/1 -> Bus Creator/23
  userDE1/1 -> Bus Creator/22
  desTrq_N_m/1 -> Bus Creator/21
  desSpeed_m_s/1 -> Bus Creator/20
  estDisLVeh_m/1 -> Bus Creator/19
  estDisPVeh_m/1 -> Bus Creator/18
  desTGapLVeh_s/1 -> Bus Creator/17
  desTGapPVeh_s/1 -> Bus Creator/16
  relSpdLVeh_m_s/1 -> Bus Creator/15
  distToLVeh_m_s/1 -> Bus Creator/14
  relSpdPVeh_m_s/1 -> Bus Creator/13
  distToPVeh_m/1 -> Bus Creator/12
  vehManID/1 -> Bus Creator/11
  vehManDes/1 -> Bus Creator/10
  vehFltMode/1 -> Bus Creator/9
  vehGrpPos/1 -> Bus Creator/8
  frntCutIn/1 -> Bus Creator/7
  vehID/1 -> Bus Creator/6
  grpManID/1 -> Bus Creator/5
  grpManDes/1 -> Bus Creator/4
  grpMode/1 -> Bus Creator/3
  grpSize/1 -> Bus Creator/2
  grpID/1 -> Bus Creator/1

== system CACC_system_struct/RTI Data/RTI Data Store/RTI Data Store/RTI Data Store ==
  RTI Data Store : Subsystem  mask(RTI_DATA_STORE){}
      mask help:
      | RTI Data Store Block. This block is used by RTI to store internal model dependent data. Deleting this block will result in data loss.
      |
      | NEVER DELETE, COPY, OR MODIFY THIS BLOCK!
      mask Help:
      | RTI Data Store Block. This block is used by RTI to store internal model dependent data. Deleting this block will result in data loss.
      | 
      | NEVER DELETE, COPY, OR MODIFY THIS BLOCK!
      mask Display: text(0.5, 0.5, ' ', 'HorizontalAlignment', 'center');

== system CACC_system_struct/RTI Data/RTI Data Store/RTI Data Store/RTI Data Store/RTI Data Store ==
